simulink model "Springs"  (R2016a)
settings: Solver=ode1  StartTime=0.0  StopTime=10  FixedStep=0.001  RelTol=1e-3
InitFcn:
  | m=0.2 % mass in kg
  | g=9.81 % gravity constant
model workspace (MAT data in the model file):
  C = 1
  D = 1
  g = 10
  m = 0.2
settings Model: Creator=chris.barlow  LastModifiedBy=chris.barlow

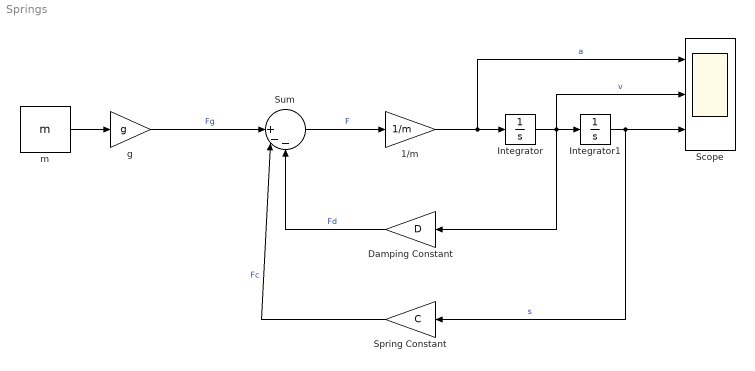
== system Springs ==
  1/m : Gain  Gain=1/m
  Damping Constant : Gain  Gain=D
  Integrator : Integrator
  Integrator1 : Integrator
      settings: AttributesFormatString=s0 = %<InitialCondition>
  Scope : Scope  NumInputPorts=3
  Spring Constant : Gain  Gain=C
  Sum : Sum  Inputs=||+--
  g : Gain  Gain=g
  m : Constant  Value=m
  wires:
  m/1 -> g/1
  g/1 -> Sum/1  "Fg"
  1/m/1 -> Scope/1, Integrator/1  "a"
  Integrator/1 -> Damping Constant/1, Scope/2, Integrator1/1  "v"
  Integrator1/1 -> Spring Constant/1, Scope/3  "s"
  Sum/1 -> 1/m/1  "F"
  Spring Constant/1 -> Sum/2  "Fc"
  Damping Constant/1 -> Sum/3  "Fd"
